simulink model "ekmsl"  (R2018a)
settings: Solver=VariableStepAuto  StartTime=0.0  StopTime=2.5  MaxStep=100e-6  RelTol=1e-3
undefined symbols (not defined in the file or in its folder): EKM
settings Model: Creator=Szalay  LastModifiedBy=Szalay

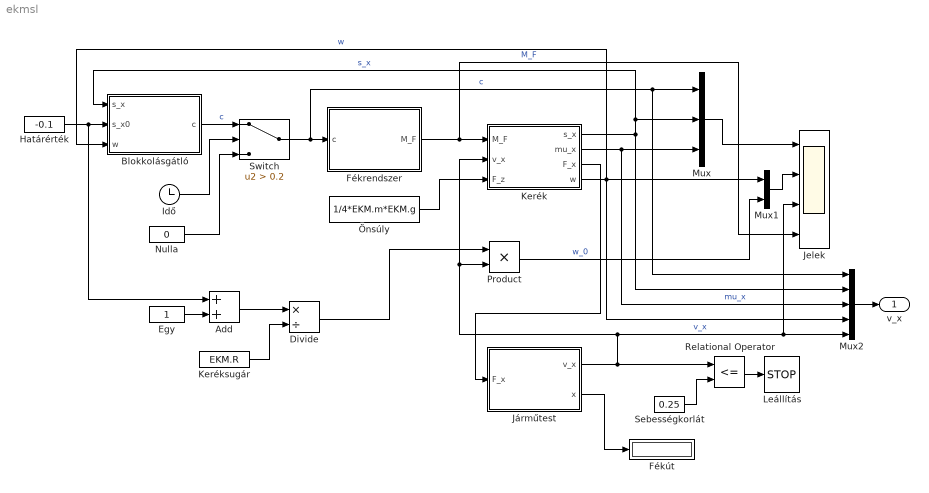
== system ekmsl ==
  Add : Sum
  Blokkolásgátló : Subsystem
  Divide : Product  Inputs=*/
  Egy : Constant
  Fékrendszer : Subsystem
  Fékút : Display
  Határérték : Constant  Value=-0.1
  Idő : Clock
  Jelek : Scope  NumInputPorts=4
  Járműtest : Subsystem
  Kerék : Subsystem
  Keréksugár : Constant  Value=EKM.R
  Leállítás : Stop
  Mux : Mux  Inputs=3
  Mux1 : Mux  Inputs=2
  Mux2 : Mux  Inputs=5
  Nulla : Constant  Value=0
  Product : Product
  Relational Operator : RelationalOperator  Operator=<=  OutDataTypeStr=boolean  RndMeth=Simplest
  Sebességkorlát : Constant  Value=0.25
  Switch : Switch  Criteria=u2 > Threshold  Threshold=0.2
  Önsúly : Constant  Value=1/4*EKM.m*EKM.g
  v_x : Outport
  wires:
  Járműtest/1(v_x) -> Relational Operator/1, Kerék/2(v_x), Product/2, Jelek/3, Mux2/5  "v_x"
  Önsúly/1 -> Kerék/3(F_z)
  Kerék/2(mu_x) -> Mux/3, Mux2/3  "mu_x"
  Kerék/1(s_x) -> Mux2/2, Blokkolásgátló/1(s_x), Mux/2  "s_x"
  Mux/1 -> Jelek/1
  Kerék/4(w) -> Mux1/1, Blokkolásgátló/3(w), Mux2/4  "w"
  Fékrendszer/1(M_F) -> Jelek/4, Kerék/1(M_F)  "M_F"
  Sebességkorlát/1 -> Relational Operator/2
  Relational Operator/1 -> Leállítás/1
  Járműtest/2(x) -> Fékút/1
  Switch/1 -> Mux/1, Mux2/1, Fékrendszer/1(c)  "c"
  Határérték/1 -> Add/1, Blokkolásgátló/2(s_x0)
  Mux1/1 -> Jelek/2
  Egy/1 -> Add/2
  Add/1 -> Divide/1
  Keréksugár/1 -> Divide/2
  Divide/1 -> Product/1
  Product/1 -> Mux1/2  "w_0"
  Kerék/3(F_x) -> Járműtest/1(F_x)
  Mux2/1 -> v_x/1
  Blokkolásgátló/1(c) -> Switch/1  "c"
  Nulla/1 -> Switch/3
  Idő/1 -> Switch/2

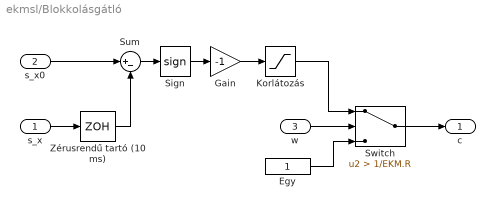
== system ekmsl/Blokkolásgátló ==
  s_x : Inport
  s_x0 : Inport  Port=2
  w : Inport  Port=3
  Egy : Constant
  Gain : Gain  Gain=-1
  Korlátozás : Saturate  UpperLimit=1  LowerLimit=0
  Sign : Signum
  Sum : Sum  Inputs=|+-
  Switch : Switch  Criteria=u2 > Threshold  Threshold=1/EKM.R
  Zérusrendű tartó (10 ms) : ZeroOrderHold  SampleTime=10e-3
  c : Outport
  wires:
  s_x/1 -> Zérusrendű tartó (10 ms)/1
  Sum/1 -> Sign/1
  Sign/1 -> Gain/1
  Gain/1 -> Korlátozás/1
  Zérusrendű tartó (10 ms)/1 -> Sum/2
  s_x0/1 -> Sum/1
  w/1 -> Switch/2
  Korlátozás/1 -> Switch/1
  Switch/1 -> c/1
  Egy/1 -> Switch/3

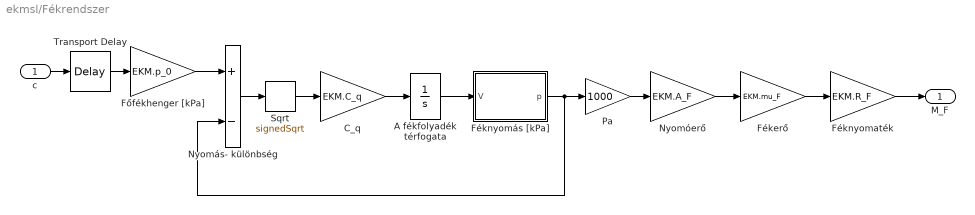
== system ekmsl/Fékrendszer ==
  c : Inport
  A fékfolyadék térfogata : Integrator  LimitOutput=on  UpperSaturationLimit=Inf  LowerSaturationLimit=0
  C_q : Gain  Gain=EKM.C_q
  Fékerő : Gain  Gain=EKM.mu_F
  Féknyomaték : Gain  Gain=EKM.R_F
  Féknyomás [kPa] : MATLAB Function  TreatAsAtomicUnit=on
  Főfékhenger [kPa] : Gain  Gain=EKM.p_0
  Nyomás- különbség : Sum  Inputs=+-
  Nyomóerő : Gain  Gain=EKM.A_F
  Pa : Gain  Gain=1000
  Sqrt : Sqrt  Operator=signedSqrt  SaturateOnIntegerOverflow=on
  Transport Delay : TransportDelay  DelayTime=EKM.T_H
  M_F : Outport
  wires:
  c/1 -> Transport Delay/1
  Transport Delay/1 -> Főfékhenger [kPa]/1
  Főfékhenger [kPa]/1 -> Nyomás- különbség/1
  Nyomás- különbség/1 -> Sqrt/1
  Sqrt/1 -> C_q/1
  C_q/1 -> A fékfolyadék térfogata/1
  A fékfolyadék térfogata/1 -> Féknyomás [kPa]/1(V)
  Féknyomás [kPa]/1(p) -> Pa/1, Nyomás- különbség/2
  Pa/1 -> Nyomóerő/1
  Nyomóerő/1 -> Fékerő/1
  Fékerő/1 -> Féknyomaték/1
  Féknyomaték/1 -> M_F/1

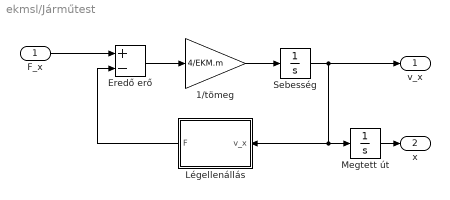
== system ekmsl/Járműtest ==
  F_x : Inport
  1/tömeg : Gain  Gain=4/EKM.m
  Eredő erő : Sum  Inputs=+-
  Légellenállás : MATLAB Function  TreatAsAtomicUnit=on
  Megtett út : Integrator  InitialCondition=EKM.v_0
  Sebesség : Integrator  InitialCondition=EKM.v_0
  v_x : Outport
  x : Outport  Port=2
  wires:
  1/tömeg/1 -> Sebesség/1
  Eredő erő/1 -> 1/tömeg/1
  Sebesség/1 -> v_x/1, Megtett út/1, Légellenállás/1(v_x)
  Légellenállás/1(F) -> Eredő erő/2
  F_x/1 -> Eredő erő/1
  Megtett út/1 -> x/1

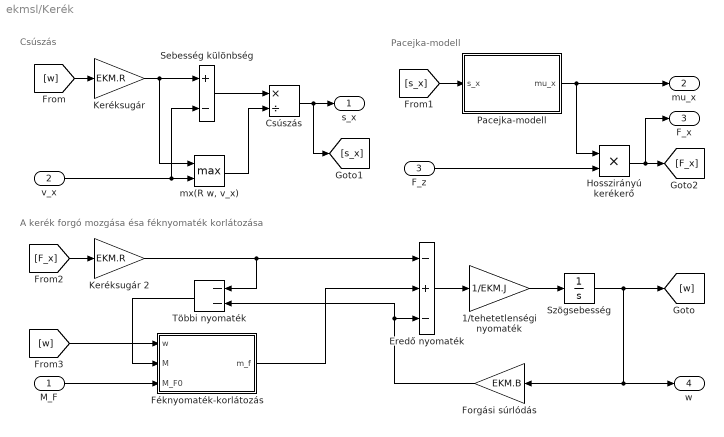
== system ekmsl/Kerék ==
  note: A kerék forgó mozgása ésa féknyomaték korlátozása
  note: Pacejka-modell
  note: Csúszás
  M_F : Inport
  v_x : Inport  Port=2
  F_z : Inport  Port=3
  1/tehetetlenségi nyomaték : Gain  Gain=1/EKM.J
  Csúszás : Product  Inputs=*/
  Eredő nyomaték : Sum  Inputs=-+-
  Forgási súrlódás : Gain  Gain=EKM.B
  Féknyomaték-korlátozás : MATLAB Function  TreatAsAtomicUnit=on
  Hosszirányú kerékerő : Product
  Keréksugár : Gain  Gain=EKM.R
  Keréksugár 2 : Gain  Gain=EKM.R
  Pacejka-modell : MATLAB Function  TreatAsAtomicUnit=on
  Sebesség különbség : Sum  Inputs=+-
  Szögsebesség : Integrator  InitialCondition=EKM.w_0  LimitOutput=on  LowerSaturationLimit=0
  Többi nyomaték : Sum  Inputs=--
  "mx(R w, v_x)" : MinMax  Function=max  Inputs=2
  s_x : Outport
  mu_x : Outport  Port=2
  F_x : Outport  Port=3
  w : Outport  Port=4
  wires:
  1/tehetetlenségi nyomaték/1 -> Szögsebesség/1
  Eredő nyomaték/1 -> 1/tehetetlenségi nyomaték/1
  Szögsebesség/1 -> [w], Forgási súrlódás/1, w/1
  Forgási súrlódás/1 -> Többi nyomaték/2, Eredő nyomaték/3
  [w] -> Keréksugár/1
  Keréksugár/1 -> "mx(R w, v_x)"/1, Sebesség különbség/1
  v_x/1 -> "mx(R w, v_x)"/2, Sebesség különbség/2
  Sebesség különbség/1 -> Csúszás/1
  "mx(R w, v_x)"/1 -> Csúszás/2
  Csúszás/1 -> [s_x], s_x/1
  [s_x] -> Pacejka-modell/1(s_x)
  Pacejka-modell/1(mu_x) -> mu_x/1, Hosszirányú kerékerő/1
  F_z/1 -> Hosszirányú kerékerő/2
  Hosszirányú kerékerő/1 -> F_x/1, [F_x]
  [F_x] -> Keréksugár 2/1
  Keréksugár 2/1 -> Többi nyomaték/1, Eredő nyomaték/1
  M_F/1 -> Féknyomaték-korlátozás/3(M_F0)
  [w] -> Féknyomaték-korlátozás/1(w)
  Féknyomaték-korlátozás/1(m_f) -> Eredő nyomaték/2
  Többi nyomaték/1 -> Féknyomaték-korlátozás/2(M)

== matlab function ekmsl/Kerék/Pacejka-modell ==
  data: s_x input; mu_x output
function mu_x = Pacejka(s_x)

mu_x = EKM.Pacejka(s_x);

end

== matlab function ekmsl/Járműtest/Légellenállás ==
  data: v_x input; F output
function F = F_L(v_x)
	
% Légellenállás
F = 1/2 * EKM.c_W * EKM.rho * EKM.A * v_x^2;

end

== matlab function ekmsl/Kerék/Féknyomaték-korlátozás ==
  data: w input; m_f output; M input; M_F0 input
function m_f = M_F(w, M, M_F0)

m_f = EKM.M_F(w, M, M_F0);

end

== matlab function ekmsl/Fékrendszer/Féknyomás [kPa] ==
  data: V input; p output
function p = F(V)

p = EKM.F(V);

end
